simulink model "Ass3"  (R2024b)
settings: Solver=FixedStepAuto  StartTime=0.0  StopTime=inf  FixedStep=1/f_sim  RelTol=1e-3
model workspace (MAT data in the model file):
  SL_ROS_VariableLengthArrays_MaxSizes.CommonInfo.ArrayTruncateAction = 'EmitWarning'
  SL_ROS_VariableLengthArrays_MaxSizes.MsgTypeMap = containers.Map
  SL_ROS_VariableLengthArrays_MaxSizes.MsgTypeMap.serialization.keys = {'sensor_msgs/Image', 'sensor_msgs/LaserScan'}
  SL_ROS_VariableLengthArrays_MaxSizes.MsgTypeMap.serialization.values{1}(1).PropertyName = 'Data'
  SL_ROS_VariableLengthArrays_MaxSizes.MsgTypeMap.serialization.values{1}(1).DataType = 'uint8'
  SL_ROS_VariableLengthArrays_MaxSizes.MsgTypeMap.serialization.values{1}(1).MaxLength = 921600
  SL_ROS_VariableLengthArrays_MaxSizes.MsgTypeMap.serialization.values{1}(2).PropertyName = 'Encoding'
  SL_ROS_VariableLengthArrays_MaxSizes.MsgTypeMap.serialization.values{1}(2).DataType = 'uint8'
  SL_ROS_VariableLengthArrays_MaxSizes.MsgTypeMap.serialization.values{1}(2).MaxLength = 128
  SL_ROS_VariableLengthArrays_MaxSizes.MsgTypeMap.serialization.values{2}(1).PropertyName = 'Intensities'
  SL_ROS_VariableLengthArrays_MaxSizes.MsgTypeMap.serialization.values{2}(1).DataType = 'single'
  SL_ROS_VariableLengthArrays_MaxSizes.MsgTypeMap.serialization.values{2}(1).MaxLength = 360
  SL_ROS_VariableLengthArrays_MaxSizes.MsgTypeMap.serialization.values{2}(2).PropertyName = 'Ranges'
  SL_ROS_VariableLengthArrays_MaxSizes.MsgTypeMap.serialization.values{2}(2).DataType = 'single'
  SL_ROS_VariableLengthArrays_MaxSizes.MsgTypeMap.serialization.values{2}(2).MaxLength = 360
  SL_ROS_VariableLengthArrays_MaxSizes.MsgTypeMap.serialization.uniformity = 0
  SL_ROS_VariableLengthArrays_MaxSizes.MsgTypeMap.serialization.keyType = 'char'
  SL_ROS_VariableLengthArrays_MaxSizes.MsgTypeMap.serialization.valueType = 'any'
values from neighbouring files (symbols this model uses):
  f_sim = 30    [Main_Ass3.m]
  scan = out.scan    [Main_Ass3.m]
  v_max = 0.26    [Main_Ass3.m]
  v_min = -0.26    [Main_Ass3.m]
  w_max = 1.82    [Main_Ass3.m]
  w_min = -1.82    [Main_Ass3.m]
undefined symbols (not defined in the file or in its folder): Angular, gray, Linear, Rec, SDTV
libraries: robotlib x6, simulink x4, visiontextngfix x2, visionconversions x1, visionstatistics x1
settings Model: Creator=vise  LastModifiedBy=vise
settings OptimizationCC: DefaultParameterBehavior=Inlined  EnhancedBackFolding=on  PassReuseOutputArgsAs=Individual arguments  ZeroExternalMemoryAtStartup=off  ZeroInternalMemoryAtStartup=off  MaxStackSize=64  OptimizeBlockOrder=speed  DifferentSizesBufferReuse=on  OptimizationCustomize=off  EfficientTunableParamExpr=on
settings DebuggingCC: ParameterTunabilityLossMsg=error
settings HardwareCC: ProdBitPerPointer=32  ProdBitPerSizeT=32  ProdBitPerPtrDiffT=32  ProdLargestAtomicFloat=None  ProdIntDivRoundTo=Undefined  ProdEndianess=Unspecified  ProdWordSize=32  ProdHWDeviceType=Generic->Unspecified (assume 32-bit Generic)  UseEmbeddedCoderFeatures=off
settings SFSimCC: MATLABDynamicMemAlloc=off
settings RTWCC: Description=Embedded Coder  SystemTargetFile=ert.tlc  HardwareBoard=Robot Operating System (ROS)  TLCOptions="-aInlineSetEventsForThisBaseRateFcn=TLC_FALSE -aSuppressMultiTaskScheduler=TLC_FALSE  -aRateBasedStepFcn=0"  TemplateMakefile=ert_default_tmf  Toolchain=Catkin  TargetLang=C++
settings CodeAppCC: ForceParamTrailComments=on  IgnoreCustomStorageClasses=off  OperatorAnnotations=on  SimulinkDataObjDesc=on  SFDataObjDesc=on  InsertBlockDesc=on
settings ERTTargetCC: SupportNonInlinedSFcns=on

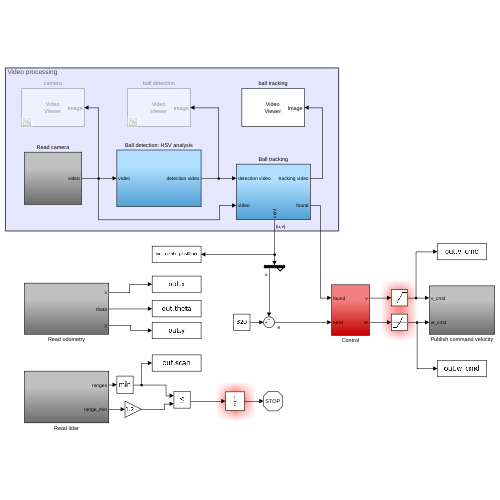
[thumbnail: Simulink's stored preview of the top-level diagram]
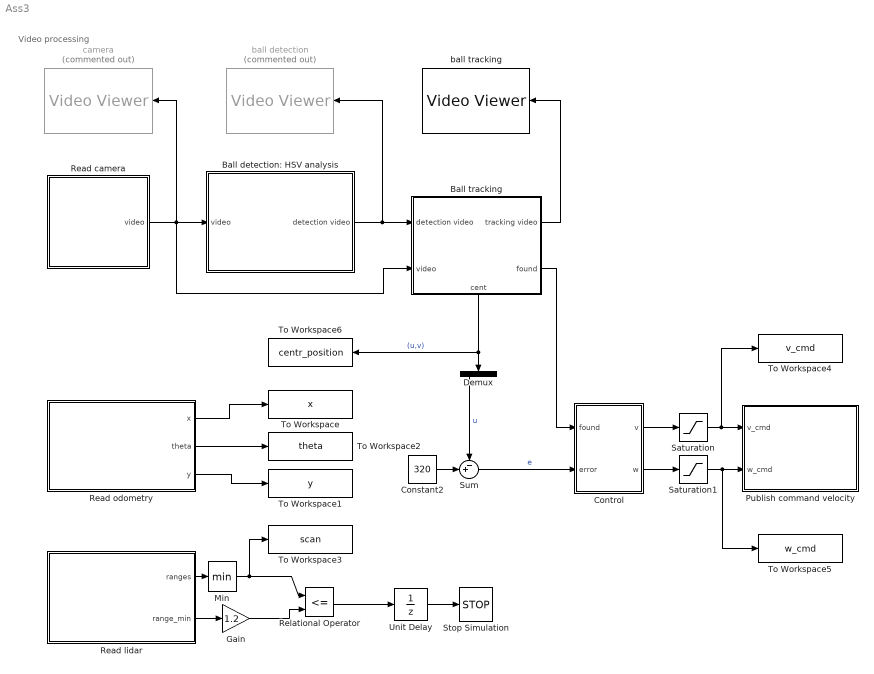
== system Ass3 ==
  note: Video processing
  Ball detection: HSV analysis : Subsystem
  Ball tracking : Subsystem
      settings: PortSchema="{\"entries\":[{\"content\":{\"sides\":[{\"content\":{\"connectorIds\":[\"In1\",\"In2\"]},\"type\":\"ConnectorPlacement.EquallySpacedRectSide\",\"uuid\":\"de28c0a8-2bee-4438-9aac-76140af63e3d\"},{\"content\":{\"connectorIds\":[\"Out1\",\"Out2\"],\"side\":\"RIGHT\"},\"type\":\"ConnectorPlacement.EquallySpacedRectSide\",\"uuid\":\"c12b1d92-09c4-48b4-970d-3ef4bedca178\"},{\"content\":{\"side\":\"TOP\"},\"type\":\"ConnectorPlacement.EquallySpacedRectSide\",\"uuid\":\"97f30cb4-6242-496e-af3a-557549f12300\"},{\"content\":{\"connectorIds\":[\"Out3\"],\"side\":\"BOTTOM\"},\"type\":\"ConnectorPlacement.EquallySpacedRectSide\",\"uuid\":\"1885ebab-ea81-4869-a630-7be10d35318a\"}]},\"type\":\"ConnectorPlacement.EquallySpacedConnector\",\"uuid\":\"dcf9ab1b-4d94-44bc-b96b-0b581f8b2e33\"}],\"packageUris\":[\"http://schema.mathworks.com/mf0/Connector/R2020b\"],\"version\":\"1.0\"}"
  Constant2 : Constant  Value=320
  Control : Subsystem
  Demux : Demux  Outputs=2
  Gain : Gain  Gain=1.2
  Min : MinMax
  Publish command velocity : Subsystem
  Read camera : Subsystem
  Read lidar : Subsystem
  Read odometry : Subsystem
  Relational Operator : RelationalOperator  Operator=<=  OutDataTypeStr=boolean  RndMeth=Simplest  InputSameDT=off
  Saturation : Saturate  UpperLimit=v_max  LowerLimit=v_min
  Saturation1 : Saturate  UpperLimit=w_max  LowerLimit=w_min
  Stop Simulation : Stop
  Sum : Sum  Inputs=-+|
  To Workspace : ToWorkspace  VariableName=x  SampleTime=-1
      settings: Save2DSignal=2-D array (concatenate along first dimension)
  To Workspace1 : ToWorkspace  VariableName=y  SampleTime=-1
      settings: Save2DSignal=2-D array (concatenate along first dimension)
  To Workspace2 : ToWorkspace  VariableName=theta  SampleTime=-1
      settings: Save2DSignal=2-D array (concatenate along first dimension)
  To Workspace3 : ToWorkspace  VariableName=scan  SampleTime=-1
      settings: Save2DSignal=2-D array (concatenate along first dimension)
  To Workspace4 : ToWorkspace  VariableName=v_cmd  SampleTime=-1
      settings: Save2DSignal=2-D array (concatenate along first dimension)
  To Workspace5 : ToWorkspace  VariableName=w_cmd  SampleTime=-1
      settings: Save2DSignal=2-D array (concatenate along first dimension)
  To Workspace6 : ToWorkspace  VariableName=centr_position  SampleTime=-1
      settings: Save2DSignal=2-D array (concatenate along first dimension)
  Unit Delay : UnitDelay  SampleTime=30*1/f_sim  HasFrameUpgradeWarning=on
  ball detection : VideoViewer  Commented=on  colormapValue=gray(256)  FigPos=[741 775 418 304]  OpenAtMdlStart=off
  ball tracking : VideoViewer  colormapValue=gray(256)  FigPos=[30 943 713 468]
  camera : VideoViewer  Commented=on  colormapValue=gray(256)  FigPos=[384 710 438 290]  OpenAtMdlStart=off
  wires:
  Read camera/1(video) -> camera/1, Ball detection: HSV analysis/1(video), Ball tracking/2(video)
  Saturation1/1 -> To Workspace5/1, Publish command velocity/2(w_cmd)
  Saturation/1 -> To Workspace4/1, Publish command velocity/1(v_cmd)
  Ball detection: HSV analysis/1(detection video) -> ball detection/1, Ball tracking/1(detection video)
  Ball tracking/1(tracking video) -> ball tracking/1
  Ball tracking/3(cent) -> To Workspace6/1, Demux/1  "(u,v)"
  Ball tracking/2(found) -> Control/1(found)
  Sum/1 -> Control/2(error)  "e"
  Control/1(v) -> Saturation/1
  Control/2(w) -> Saturation1/1
  Constant2/1 -> Sum/2
  Demux/1 -> Sum/1  "u"
  Read odometry/1(x) -> To Workspace/1
  Read odometry/2(theta) -> To Workspace2/1
  Read odometry/3(y) -> To Workspace1/1
  Min/1 -> Relational Operator/1, To Workspace3/1
  Read lidar/1(ranges) -> Min/1
  Read lidar/2(range_min) -> Gain/1
  Gain/1 -> Relational Operator/2
  Relational Operator/1 -> Unit Delay/1
  Unit Delay/1 -> Stop Simulation/1

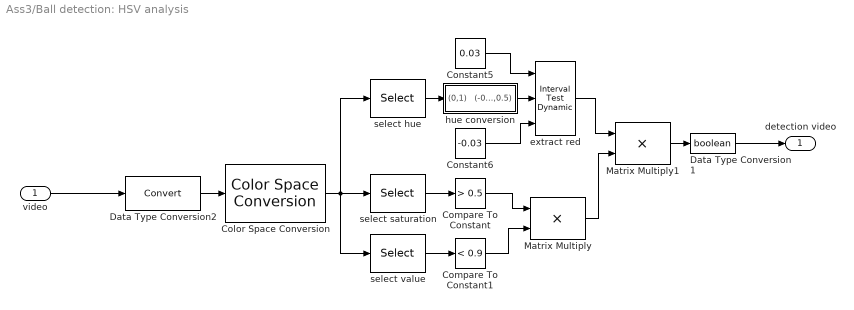
== system Ass3/Ball detection: HSV analysis ==
  video : Inport
  Color Space Conversion : visionconversions/Color Space  Conversion  conversion=Obsolete  conversionActive=R'G'B' to HSV  wp_str=D65  rec=Rec. 601 (SDTV)  sys=1125/60/2:1  imagePorts=One multidimensional signal
  Compare To Constant : simulink/Logic and Bit Operations/Compare To Constant  relop=>  const=0.5  OutDataTypeStr=boolean
  Compare To Constant1 : simulink/Logic and Bit Operations/Compare To Constant  relop=<  const=0.9  OutDataTypeStr=boolean
  Constant5 : Constant  Value=0.03
  Constant6 : Constant  Value=-0.03
  Data Type Conversion1 : DataTypeConversion  OutDataTypeStr=boolean  SaturateOnIntegerOverflow=off  RndMeth=Floor
  Data Type Conversion2 : DataTypeConversion  SaturateOnIntegerOverflow=off  RndMeth=Floor
  Matrix Multiply : Product
  Matrix Multiply1 : Product
  extract red : simulink/Logic and Bit Operations/Interval Test Dynamic  IntervalClosedRight=on  IntervalClosedLeft=on  OutDataTypeStr=boolean
  hue conversion : Subsystem
  select hue : Selector  NumberOfDimensions=3  InputPortWidth=3  IndexOptions=Select all,Select all,Index vector (dialog)  Indices=[1 3],1,1  OutputSizes=1,1,1
  select saturation : Selector  NumberOfDimensions=3  InputPortWidth=3  IndexOptions=Select all,Select all,Index vector (dialog)  Indices=[1 3],1,2  OutputSizes=1,1,1
  select value : Selector  NumberOfDimensions=3  InputPortWidth=3  IndexOptions=Select all,Select all,Index vector (dialog)  Indices=[1 3],1,2  OutputSizes=1,1,1
  detection video : Outport
  wires:
  Constant6/1 -> extract red/3
  Matrix Multiply/1 -> Matrix Multiply1/2
  video/1 -> Data Type Conversion2/1
  extract red/1 -> Matrix Multiply1/1
  Compare To Constant1/1 -> Matrix Multiply/2
  Color Space Conversion/1 -> select value/1, select saturation/1, select hue/1
  select value/1 -> Compare To Constant1/1
  Data Type Conversion1/1 -> detection video/1
  Data Type Conversion2/1 -> Color Space Conversion/1
  Matrix Multiply1/1 -> Data Type Conversion1/1
  Compare To Constant/1 -> Matrix Multiply/1
  hue conversion/1((-0.5,0.5)) -> extract red/2
  Constant5/1 -> extract red/1
  select saturation/1 -> Compare To Constant/1
  select hue/1 -> hue conversion/1((0,1))

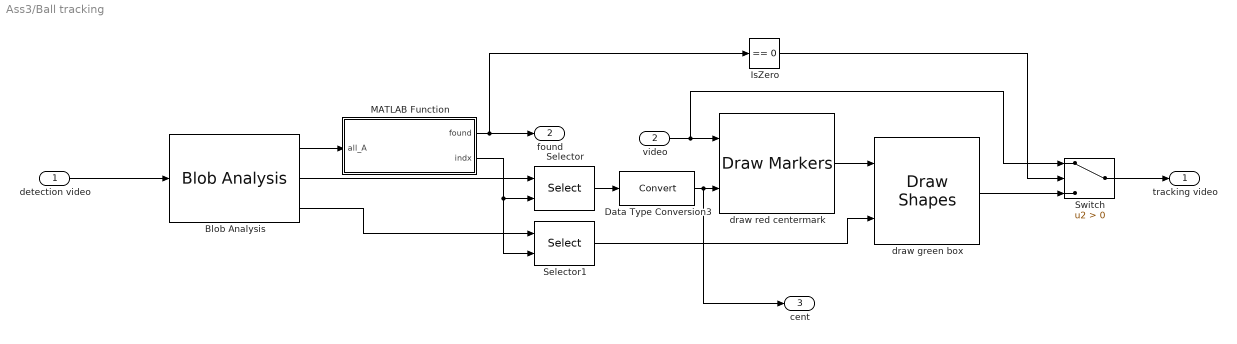
== system Ass3/Ball tracking ==
  detection video : Inport
  video : Inport  Port=2
  Blob Analysis : visionstatistics/Blob Analysis  Tag=vipblks_row_conv  area=on  centroid=on  bBox=on  majorAxis=off  minorAxis=off  angle=off  eccentricity=off  equivDiameterSq=off  extent=off  perimeter=off  outDT=double  conn=8  isLabel=off  maxBlobs=5  warnIfNumBlobsExceeded=on  isCount=off  useMinArea=off  minArea=0  useMaxArea=off  maxArea=intmax('uint32')  excludeBorderBlob=off  isOutVarDim=off  isFill=on  fillValues=-1  roundingMode=Floor  overflowMode=off  prodOutputMode=Binary point scaling  prodOutputWordLength=32  prodOutputFracLength=16  accumMode=Binary point scaling  accumWordLength=32  accumFracLength=0  outputMode=Binary point scaling  outputWordLength=32  outputFracLength=16  firstCoeffMode=Binary point scaling  firstCoeffWordLength=16  firstCoeffFracLength=14  secondCoeffMode=Binary point scaling  secondCoeffWordLength=32  secondCoeffFracLength=16
  Data Type Conversion3 : DataTypeConversion  SaturateOnIntegerOverflow=off  RndMeth=Floor
  IsZero : simulink/Logic and Bit Operations/Compare To Zero  relop===  OutDataTypeStr=boolean
      settings: LibrarySourceBlock=|
      | simulink/Quick Insert/Logic and Bit
      | Operations/IsZero
  MATLAB Function : MATLAB Function  TreatAsAtomicUnit=on
  Selector : Selector  NumberOfDimensions=2  InputPortWidth=3  IndexOptions=Index vector (port),Select all  Indices=[1 3],1  OutputSizes=1,1
  Selector1 : Selector  NumberOfDimensions=2  InputPortWidth=3  IndexOptions=Index vector (port),Select all  Indices=[1 3],1  OutputSizes=1,1
  Switch : Switch  Criteria=u2 > Threshold  SaturateOnIntegerOverflow=off  InputSameDT=off
  draw green box : visiontextngfix/Draw Shapes  shape=Rectangles  fill=off  lineWidth=1  fillClrSource=Specify via dialog  display=User-specified value  intensity=200  color=[0 255 0]  opacity=0.6  viewport=Entire image  antialiasing=off  inType=Obsolete  imagePorts=One multidimensional signal  roundingMode=Floor  overflowMode=off  memoryMode=Specify word length  memoryWordLength=16  prodOutputMode=Binary point scaling  prodOutputWordLength=32  prodOutputFracLength=14  memoryFracLength=15
  draw red centermark : visiontextngfix/Draw Markers  shape=Plus  size=3  fill=off  fillClrSource=Specify via dialog  display=User-specified value  intensity=200  color=[255 0 0]  opacity=0.6  viewport=Entire image  antialiasing=off  inType=Obsolete  imagePorts=One multidimensional signal  roundingMode=Floor  overflowMode=off  memoryMode=Specify word length  memoryWordLength=16  memoryFracLength=15  prodOutputMode=Binary point scaling  prodOutputWordLength=32  prodOutputFracLength=14
  tracking video : Outport
  found : Outport  Port=2
  cent : Outport  Port=3
  wires:
  Blob Analysis/1 -> MATLAB Function/1(all_A)
  Data Type Conversion3/1 -> cent/1, draw red centermark/2
  detection video/1 -> Blob Analysis/1
  Selector1/1 -> draw green box/2
  draw green box/1 -> Switch/3
  draw red centermark/1 -> draw green box/1
  Blob Analysis/3 -> Selector1/1
  MATLAB Function/2(indx) -> Selector1/2, Selector/2
  Blob Analysis/2 -> Selector/1
  Switch/1 -> tracking video/1
  Selector/1 -> Data Type Conversion3/1
  MATLAB Function/1(found) -> found/1, IsZero/1
  video/1 -> Switch/1, draw red centermark/1
  IsZero/1 -> Switch/2

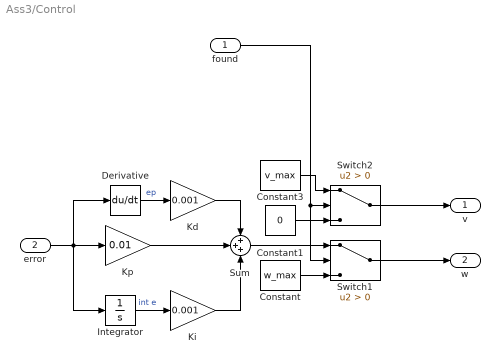
== system Ass3/Control ==
  found : Inport
  error : Inport  Port=2
  Constant : Constant  Value=w_max
  Constant1 : Constant  Value=0
  Constant3 : Constant  Value=v_max
  Derivative : Derivative
  Integrator : Integrator
  Kd : Gain  Gain=0.001
  Ki : Gain  Gain=0.001
  Kp : Gain  Gain=0.01
  Sum : Sum  Inputs=+++
  Switch1 : Switch  Criteria=u2 > Threshold  SaturateOnIntegerOverflow=off  InputSameDT=off
  Switch2 : Switch  Criteria=u2 > Threshold  SaturateOnIntegerOverflow=off  InputSameDT=off
  v : Outport
  w : Outport  Port=2
  wires:
  error/1 -> Derivative/1, Kp/1, Integrator/1
  Kp/1 -> Sum/2
  Switch1/1 -> w/1
  Constant3/1 -> Switch2/1
  Switch2/1 -> v/1
  Constant1/1 -> Switch2/3
  Constant/1 -> Switch1/3
  found/1 -> Switch1/2, Switch2/2
  Derivative/1 -> Kd/1  "ep"
  Sum/1 -> Switch1/1
  Kd/1 -> Sum/1
  Integrator/1 -> Ki/1  "int e"
  Ki/1 -> Sum/3

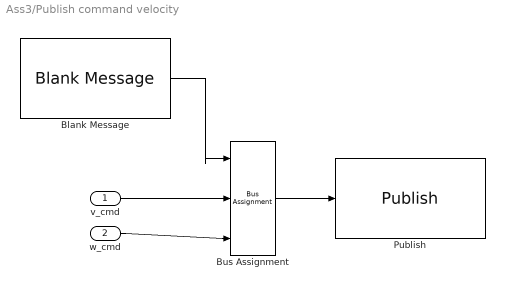
== system Ass3/Publish command velocity ==
  v_cmd : Inport
  w_cmd : Inport  Port=2
  Blank Message : robotlib/Blank Message  messageClass=Message  entityType=geometry_msgs/Twist  messageType=geometry_msgs/Twist  SampleTime=1/f_sim  legacyBusStruct=off
  Bus Assignment : BusAssignment  AssignedSignals=Linear.X,Angular.Z
  Publish : robotlib/Publish  topicSource=Select from ROS network  topic=/cmd_vel  messageType=geometry_msgs/Twist  legacyBusStruct=off  messageQueueLength=1
  wires:
  Bus Assignment/1 -> Publish/1
  w_cmd/1 -> Bus Assignment/3
  Blank Message/1 -> Bus Assignment/1
  v_cmd/1 -> Bus Assignment/2

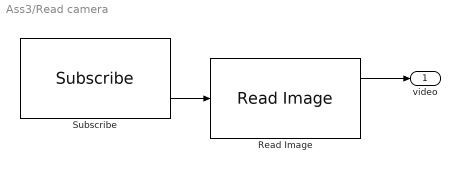
== system Ass3/Read camera ==
  Read Image : robotlib/Read Image  MaximumImageSize=[480, 640]  ImageEncoding=rgb8  ShowAlphaOutput=off  ShowErrorCodeOutput=on  VariableSizeOutputs=off
  Subscribe : robotlib/Subscribe  topicSource=Select from ROS network  topic=/camera/rgb/image_raw  messageType=sensor_msgs/Image  SampleTime=1/f_sim  legacyBusStruct=off  messageQueueLength=1
  video : Outport
  wires:
  Subscribe/2 -> Read Image/1
  Read Image/1 -> video/1

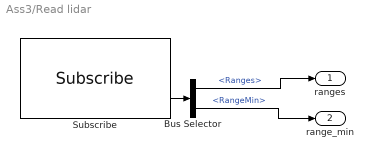
== system Ass3/Read lidar ==
  Bus Selector : BusSelector  OutputSignals=Ranges,RangeMin
  Subscribe : robotlib/Subscribe  topicSource=Select from ROS network  topic=/scan  messageType=sensor_msgs/LaserScan  SampleTime=1/f_sim  legacyBusStruct=off  messageQueueLength=1
  ranges : Outport
  range_min : Outport  Port=2
  wires:
  Subscribe/2 -> Bus Selector/1
  Bus Selector/1 -> ranges/1  "<Ranges>"
  Bus Selector/2 -> range_min/1  "<RangeMin>"

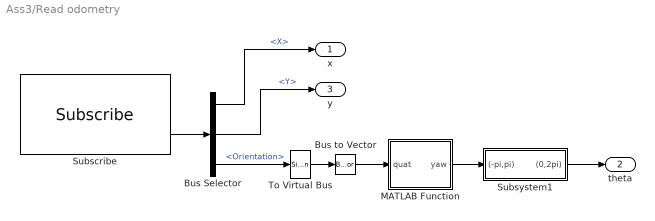
== system Ass3/Read odometry ==
  Bus Selector : BusSelector  OutputSignals=Pose.Pose.Position.X,Pose.Pose.Position.Y,Pose.Pose.Orientation
  Bus to Vector : BusToVector
  MATLAB Function : MATLAB Function  TreatAsAtomicUnit=on
  Subscribe : robotlib/Subscribe  topicSource=Select from ROS network  topic=/odom  messageType=nav_msgs/Odometry  SampleTime=1/f_sim  legacyBusStruct=off  messageQueueLength=1
  Subsystem1 : Subsystem
  To Virtual Bus : SignalConversion  ConversionOutput=Virtual bus  OverrideOpt=off
  x : Outport
  theta : Outport  Port=2
  y : Outport  Port=3
  wires:
  Subscribe/2 -> Bus Selector/1
  Bus to Vector/1 -> MATLAB Function/1(quat)
  Bus Selector/3 -> To Virtual Bus/1  "<Orientation>"
  Subsystem1/1((0,2pi)) -> theta/1
  Bus Selector/2 -> y/1  "<Y>"
  Bus Selector/1 -> x/1  "<X>"
  MATLAB Function/1(yaw) -> Subsystem1/1((-pi,pi))
  To Virtual Bus/1 -> Bus to Vector/1

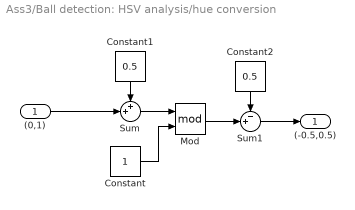
== system Ass3/Ball detection: HSV analysis/hue conversion ==
  (0,1) : Inport
  Constant : Constant
  Constant1 : Constant  Value=0.5
  Constant2 : Constant  Value=0.5
  Mod : Math  Operator=mod
  Sum : Sum  Inputs=++|
  Sum1 : Sum  Inputs=-+|
  (-0.5,0.5) : Outport
  wires:
  Constant1/1 -> Sum/1
  Constant/1 -> Mod/2
  Sum/1 -> Mod/1
  Sum1/1 -> (-0.5,0.5)/1
  (0,1)/1 -> Sum/2
  Mod/1 -> Sum1/2
  Constant2/1 -> Sum1/1

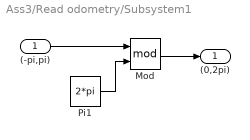
== system Ass3/Read odometry/Subsystem1 ==
  (-pi,pi) : Inport
  Mod : Math  Operator=mod
  Pi1 : Constant  Value=2*pi  OutDataTypeStr=Inherit: Inherit via back propagation
  (0,2pi) : Outport
  wires:
  (-pi,pi)/1 -> Mod/1
  Pi1/1 -> Mod/2
  Mod/1 -> (0,2pi)/1

== matlab function Ass3/Ball tracking/MATLAB Function ==
  data: found output; all_A input; indx output
function [found,indx]=FindMaxArea(all_A)

[max_A,indx]=max(all_A);

if isempty(indx) || max_A==-1
    found=0;
else
    found=1;
end

end

== matlab function Ass3/Read odometry/MATLAB Function ==
  data: quat input; yaw output
function yaw=quat2yaw(quat)

q=zeros(1,4);

q(1)=quat(1);
q(2)=quat(2);
q(3)=quat(3);
q(4)=quat(4);

eul=quat2eul(q);

yaw=eul(3);

end
